simulink model "backstepping_ceilground"  (R2025a)
settings: Solver=VariableStepAuto  StartTime=0.0  StopTime=t_total(end)  RelTol=1e-3
StopFcn:
  | autoplot;
values from neighbouring files (symbols this model uses):
  Ib = diag([params.Ix, params.Iy, params.Iz])    [setup_mission.m]
  lin_vel_0 = [0; 0; 0]    [setup_mission.m]
  mass = params.m    [setup_mission.m]
  pos_0 = p_ref(:,1) + offset_init    [setup_mission.m]
  w_bb_0 = [0; 0; 0]    [setup_mission.m]
libraries: robotcorelib x2, uavutilslib x1
settings Model: Creator=marco  LastModifiedBy=marco

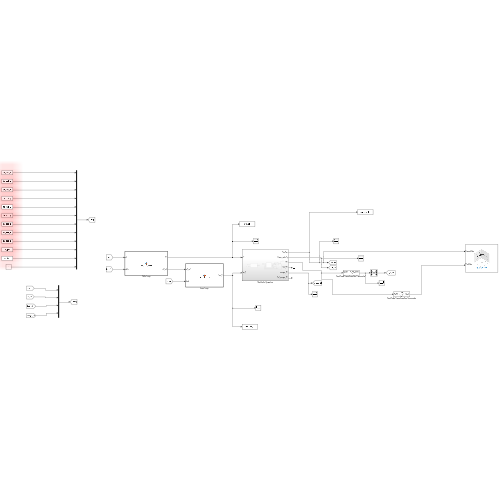
[thumbnail: Simulink's stored preview of the top-level diagram]
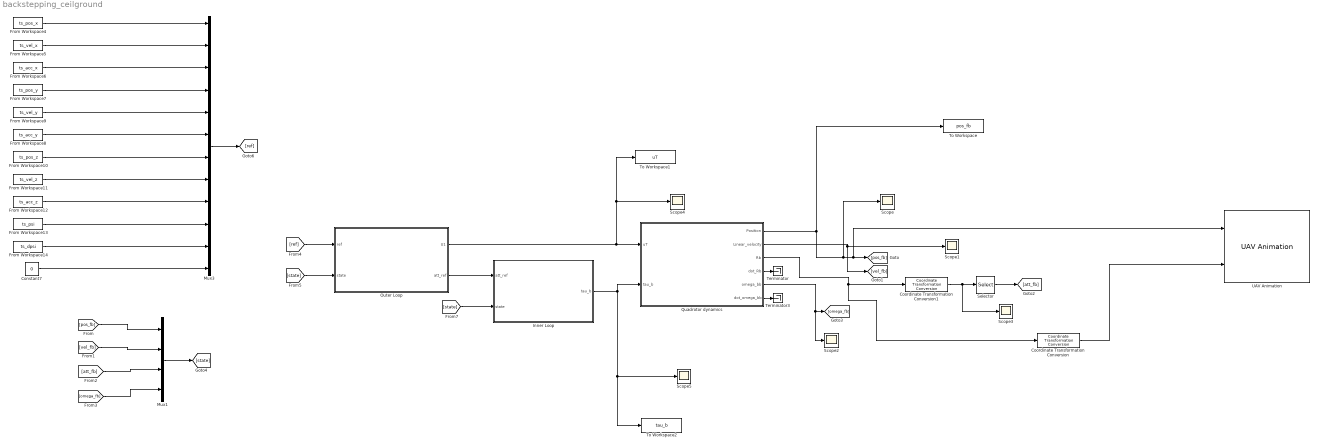
== system backstepping_ceilground ==
  Constant7 : Constant  Value=0
  Coordinate Transformation Conversion : robotcorelib/Coordinate Transformation Conversion  InputRepresentation=Rotation Matrix  InputEulerSequence=ZYX  ShowTrVecInputPort=on  OutputRepresentation=Quaternion  OutputEulerSequence=ZYX  ShowTrVecOutputPort=on  SimulateUsing=Interpreted execution
  Coordinate Transformation Conversion1 : robotcorelib/Coordinate Transformation Conversion  InputRepresentation=Rotation Matrix  InputEulerSequence=ZYX  ShowTrVecInputPort=on  OutputRepresentation=Euler Angles  OutputEulerSequence=ZYX  ShowTrVecOutputPort=on  SimulateUsing=Interpreted execution
  From Workspace10 : FromWorkspace  VariableName=ts_pos_z
  From Workspace11 : FromWorkspace  VariableName=ts_vel_z
  From Workspace12 : FromWorkspace  VariableName=ts_acc_z
  From Workspace13 : FromWorkspace  VariableName=ts_psi
  From Workspace14 : FromWorkspace  VariableName=ts_dpsi
  From Workspace4 : FromWorkspace  VariableName=ts_pos_x
  From Workspace5 : FromWorkspace  VariableName=ts_vel_x
  From Workspace6 : FromWorkspace  VariableName=ts_acc_x
  From Workspace7 : FromWorkspace  VariableName=ts_pos_y
  From Workspace8 : FromWorkspace  VariableName=ts_acc_y
  From Workspace9 : FromWorkspace  VariableName=ts_vel_y
  Inner Loop : MATLAB Function  TreatAsAtomicUnit=on
  Mux1 : Mux
  Mux3 : Mux  Inputs=12
  Outer Loop : MATLAB Function  TreatAsAtomicUnit=on
  Quadrotor dynamics : Subsystem
  Scope{,1..5} (6 alike) : Scope
      Scope settings: ActiveDisplayYMinimum=-4.6326382236688541  ActiveDisplayYMaximum=1.6258456698835591
      Scope1 settings: ActiveDisplayYMinimum=-1  ActiveDisplayYMaximum=1
      Scope2 settings: ActiveDisplayYMinimum=-1  ActiveDisplayYMaximum=1  DataLoggingVariableName=ScopeData2
      Scope3 settings: ActiveDisplayYMinimum=-1  ActiveDisplayYMaximum=1  DataLoggingVariableName=ScopeData3
      Scope4 settings: ActiveDisplayYMinimum=11.687086404838853  ActiveDisplayYMaximum=11.856708503122613  DataLoggingVariableName=ScopeData4
      Scope5 settings: ActiveDisplayYMinimum=-0.020164289135421433  ActiveDisplayYMaximum=0.020163735646024  DataLoggingVariableName=ScopeData5
  Selector : Selector  InputPortWidth=3  IndexOptions=Index vector (dialog)  Indices=[3, 2, 1]  OutputSizes=1
  Terminator : Terminator
  Terminator3 : Terminator
  To Workspace : ToWorkspace  VariableName=pos_fb  SaveFormat=Timeseries  SampleTime=-1
  To Workspace1 : ToWorkspace  VariableName=uT  SaveFormat=Timeseries  SampleTime=-1
  To Workspace2 : ToWorkspace  VariableName=tau_b  SaveFormat=Timeseries  SampleTime=-1
  UAV Animation : uavutilslib/UAV Animation  NumUAV=1  DynamicUAVConfig=off  UAVType=Multirotor  UAVSize=1  UAVColor=[1 0 0]  UAVTrajectoryAlpha=1  InertialZDirection=Down  RotationFormat=Quaternion  DrawMarkers=off  SampleTime=0.01
  wires:
  From Workspace5/1 -> Mux3/2
  From Workspace11/1 -> Mux3/8
  Coordinate Transformation Conversion/1 -> UAV Animation/2
  From Workspace7/1 -> Mux3/4
  From Workspace12/1 -> Mux3/9
  Constant7/1 -> Mux3/12
  From Workspace8/1 -> Mux3/6
  Mux3/1 -> [ref]
  Selector/1 -> [att_fb]
  Quadrotor dynamics/2(Linear_velocity) -> [vel_fb], Scope1/1
  From Workspace9/1 -> Mux3/5
  [vel_fb] -> Mux1/2
  Quadrotor dynamics/3(Rb) -> Coordinate Transformation Conversion/1, Coordinate Transformation Conversion1/1
  From Workspace6/1 -> Mux3/3
  From Workspace10/1 -> Mux3/7
  Quadrotor dynamics/4(dot_Rb) -> Terminator/1
  From Workspace13/1 -> Mux3/10
  [att_fb] -> Mux1/3
  Quadrotor dynamics/6(dot_omega_bb) -> Terminator3/1
  Coordinate Transformation Conversion1/1 -> Selector/1, Scope3/1
  Quadrotor dynamics/5(omega_bb) -> Scope2/1, [omega_fb]
  [pos_fb] -> Mux1/1
  From Workspace4/1 -> Mux3/1
  [omega_fb] -> Mux1/4
  From Workspace14/1 -> Mux3/11
  Quadrotor dynamics/1(Position) -> Scope/1, UAV Animation/1, [pos_fb], To Workspace/1
  Mux1/1 -> [state]
  [state] -> Outer Loop/2(state)
  [ref] -> Outer Loop/1(ref)
  Outer Loop/1(U1) -> To Workspace1/1, Scope4/1, Quadrotor dynamics/1(uT)
  Inner Loop/1(tau_b) -> To Workspace2/1, Scope5/1, Quadrotor dynamics/2(tau_b)
  [state] -> Inner Loop/2(state)
  Outer Loop/2(att_ref) -> Inner Loop/1(att_ref)

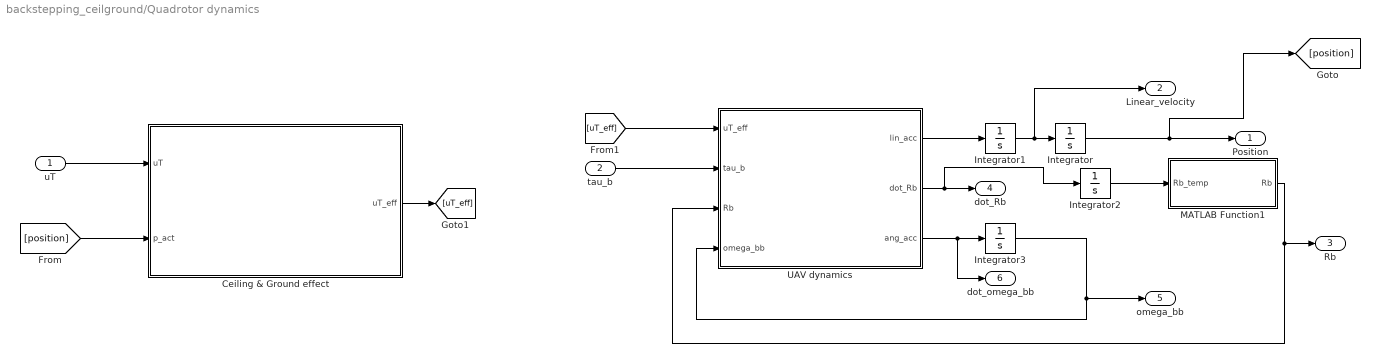
== system backstepping_ceilground/Quadrotor dynamics ==
  uT : Inport
  tau_b : Inport  Port=2
  Ceiling & Ground effect : MATLAB Function  TreatAsAtomicUnit=on
  Integrator : Integrator  InitialCondition=pos_0
  Integrator1 : Integrator  InitialCondition=lin_vel_0
  Integrator2 : Integrator  InitialCondition=[1 0 0; 0 1 0;0 0 1]
  Integrator3 : Integrator  InitialCondition=w_bb_0
  MATLAB Function1 : MATLAB Function  TreatAsAtomicUnit=on
  UAV dynamics : MATLAB Function  TreatAsAtomicUnit=on
  Position : Outport
  Linear_velocity : Outport  Port=2
  Rb : Outport  Port=3
  dot_Rb : Outport  Port=4
  omega_bb : Outport  Port=5
  dot_omega_bb : Outport  Port=6
  wires:
  Integrator/1 -> [position], Position/1
  Integrator2/1 -> MATLAB Function1/1(Rb_temp)
  UAV dynamics/1(lin_acc) -> Integrator1/1
  Integrator3/1 -> UAV dynamics/4(omega_bb), omega_bb/1
  Ceiling & Ground effect/1(uT_eff) -> [uT_eff]
  UAV dynamics/2(dot_Rb) -> Integrator2/1, dot_Rb/1
  UAV dynamics/3(ang_acc) -> dot_omega_bb/1, Integrator3/1
  Integrator1/1 -> Linear_velocity/1, Integrator/1
  MATLAB Function1/1(Rb) -> Rb/1, UAV dynamics/3(Rb)
  tau_b/1 -> UAV dynamics/2(tau_b)
  [uT_eff] -> UAV dynamics/1(uT_eff)
  uT/1 -> Ceiling & Ground effect/1(uT)
  [position] -> Ceiling & Ground effect/2(p_act)

== matlab function backstepping_ceilground/Quadrotor dynamics/Ceiling & Ground effect ==
  data: uT input; uT_eff output; p_act input
function uT_eff = aero_disturbances(uT, p_act)

% --- ENVIRONMENTAL AND DRONE PARAMETERS ---
R = 0.15;           % Propeller radius [m] (Typical OS4)
H_room = 3.0;       % Room height [m] 

% Ceiling Effect Coefficients
k1 = 6.924;
k2 = 0.03782;

% --- DISTANCES CALCULATION  ---
z_drone = p_act(3);         % Current altitude (negative in flight)
d_ground = -z_drone;        % Distance from floor (z=0)
d_ceil   = H_room - d_ground; % Distance from ceiling (z=-3)

% Safety saturation to prevent division by zero
d_ground = max(0.05, d_ground);
d_ceil   = max(0.05, d_ceil);

% --- GROUND EFFECT ---
K_ground = 1.0;
if d_ground < (2 * R)
    ratio_g = (R / (4 * d_ground))^2;
    ratio_g = min(ratio_g, 0.9); % Saturation to prevent singularities
    K_ground = 1 / (1 - ratio_g);
end

% --- CEILING EFFECT ---
K_ceil = 1.0;
if d_ceil < (2 * R)
    term_num = (R / (d_ceil + k2))^2;
    term_den = k1;
    ratio_c  = term_num / term_den;
    ratio_c  = min(ratio_c, 0.9); % Saturation
    K_ceil   = 1 / (1 - ratio_c);
end
% --- EFFECTIVE THRUST CALCULATION ---
K_tot = K_ground * K_ceil;
uT_eff = uT * K_tot;
end

== matlab function backstepping_ceilground/Outer Loop ==
  data: ref input; U1 output; state input; att_ref output; params parameter
function [U1, att_ref] = bs_outer_loop(ref, state, params)

x = state(1); y = state(2); z = state(3);
vx = state(4); vy = state(5); vz = state(6);
psi = state(9);
m = params.m; 
g = 9.81; 

x_d  = ref(1); vx_d = ref(2); ax_d = ref(3);
y_d  = ref(4); vy_d = ref(5); ay_d = ref(6);
z_d  = ref(7); vz_d = ref(8); az_d = ref(9);

psi_d   = ref(10); dpsi_d  = ref(11);
pos_d = [x_d; y_d; z_d];
vel_d = [vx_d; vy_d; vz_d];
acc_d = [ax_d; ay_d; az_d];
pos_act = [x; y; z];
vel_act = [vx; vy; vz];

% --- GAIN TUNING ---
Kp = [6.0; 6.0; 20.0];    
Kd = [4.5; 4.5; 12.0];    

% --- DESIRED FORCE CALCULATION ---
e_pos = pos_d - pos_act;
e_vel = vel_d - vel_act;

acc_des = acc_d + Kp .* e_pos + Kd .* e_vel;

% Total Inertial Force (F = m*a - m*g)
g_vec = [0; 0; g];
F_des_inertial = m * (acc_des - g_vec); 

% --- Total Thrust ---
U1 = norm(F_des_inertial);
U1 = max(1.0, min(25, U1)); % Saturation

% --- DESIRED ANGLES EXTRACTION ---
R_psi = [cos(psi) -sin(psi) 0;
         sin(psi)  cos(psi) 0;
         0         0        1];
         
F_body_intermediate = R_psi' * F_des_inertial; 
Fx_cmd = F_body_intermediate(1);
Fy_cmd = F_body_intermediate(2);

% Dynamic Inversion
theta_d = asin(-Fx_cmd / U1);
phi_d = asin(Fy_cmd / (U1 * cos(theta_d)));

% Angles Saturation (Safety ~35 degrees)
lim_ang = 0.6; 
theta_d = max(-lim_ang, min(lim_ang, theta_d));
phi_d   = max(-lim_ang, min(lim_ang, phi_d));

% Complex numbers check (safety)
if ~isreal(theta_d), theta_d = 0; end
if ~isreal(phi_d), phi_d = 0; end

% --- OUTPUT ---

att_ref = [phi_d; theta_d; psi_d; dpsi_d];
end

== matlab function backstepping_ceilground/Quadrotor dynamics/UAV dynamics ==
  data: uT_eff input size=1; tau_b input size=3; lin_acc output size=3; Rb input size=[3,3]; omega_bb input size=3; dot_Rb output size=[3,3]; ang_acc output size=3; mass parameter size=1; Ib parameter size=[3,3]
function [lin_acc, dot_Rb, ang_acc] = uav_dynamics(uT_eff, tau_b, Rb, omega_bb, mass, Ib)

% --- PARAMETRIC UNCERTAINTY ---

m_real = mass * 1.4; 
g = 9.81;
e3 = [0; 0; 1];

% --- TRANSLATIONAL DYNAMICS ---

Thrust_Inertial = (uT_eff / m_real) * Rb * e3;

lin_acc = g * e3 - Thrust_Inertial; 

% --- ROTATIONAL DYNAMICS ---
dot_Rb = Rb * skew(omega_bb);
ang_acc = Ib \ (-skew(omega_bb) * Ib * omega_bb + tau_b);
end
function S = skew(v)
if(numel(v)~= 1)
    S= [0 -v(3) v(2); v(3) 0 -v(1); -v(2) v(1) 0];
else
    S= zeros(3);
end
end

== matlab function backstepping_ceilground/Inner Loop ==
  data: att_ref input; tau_b output; state input; params parameter
function tau_b  = bs_inner_loop(att_ref, state, params)

% References from Outer Loop
phi_d  = att_ref(1);
theta_d = att_ref(2);
psi_d   = att_ref(3);
dpsi_d  = att_ref(4);

% Current state
phi = state(7); theta = state(8); psi = state(9);
p = state(10); q = state(11); r = state(12);
Ix = params.Ix; Iy = params.Iy; Iz = params.Iz;

% --- GAIN TUNING ---
K_att  = [70; 70; 40];    
K_rate = [18; 18; 14];    

% --- ATTITUDE CONTROL ---
e_phi   = phi_d - phi;
e_theta = theta_d - theta;
e_psi   = psi_d - psi;
de_phi   = 0 - p;       
de_theta = 0 - q;
de_psi   = dpsi_d - r;  

% --- CONTROL TORQUES CALCULATION ---
tau_phi   = Ix * (K_att(1) * e_phi   + K_rate(1) * de_phi);
tau_theta = Iy * (K_att(2) * e_theta + K_rate(2) * de_theta);
tau_psi   = Iz * (K_att(3) * e_psi   + K_rate(3) * de_psi);

% --- OUTPUT ---
tau_b = [tau_phi; tau_theta; tau_psi];
end

== matlab function backstepping_ceilground/Quadrotor dynamics/MATLAB Function1 ==
  data: Rb_temp input; Rb output
function Rb = fcn(Rb_temp)
    [U,S,V] = svd(Rb_temp);
    sigma = det(U*V');
    S_ = diag([1 1 sigma]);

    Rb = U*S_*V';
end
